simulink model "LQR"  (R2021b)
settings: Solver=VariableStepAuto  StartTime=0.0  StopTime=20  RelTol=1e-3
model workspace (MAT data in the model file):
  L = 0.2
values from neighbouring files (symbols this model uses):
  g = 9.81    [simConstants.m]
  K = lqr(A,B,Q,R,0)    [simConstants.m]
  theta0 = deg2rad(5)    [simConstants.m]
  Ts = 50e-6    (= 5e-05)    [simConstants.m]
libraries: simulink_extras x1
settings Model: Creator=logan  LastModifiedBy=logan

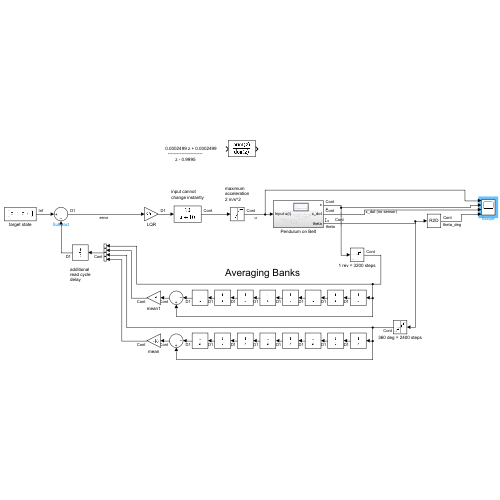
[thumbnail: Simulink's stored preview of the top-level diagram]
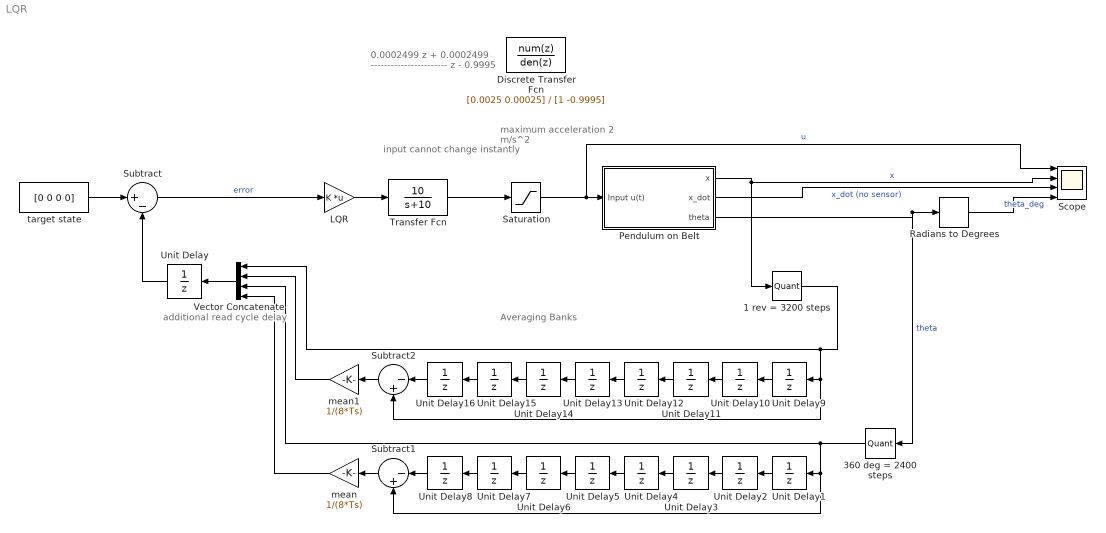
== system LQR ==
  note: 0.0002499 z + 0.0002499
      |   -----------------------
      |         z - 0.9995
  note: Averaging Banks
  note: input cannot
      | change instantly
  note: maximum
      | acceleration
      | 2 m/s^2
  note: additional
      | read cycle
      | delay
  1 rev = 3200 steps : Quantizer  QuantizationInterval=2*pi*0.006/3200
  360 deg = 2400 steps : Quantizer  QuantizationInterval=2*pi/2400
  Discrete Transfer Fcn : DiscreteTransferFcn  Numerator=[0.0025 0.00025]  Denominator=[1 -0.9995]
  LQR : Gain  Gain=K  Multiplication=Matrix(K*u)
  Pendulum on Belt : Subsystem
  Radians to Degrees : simulink_extras/Transformations/Radians to Degrees
  Saturation : Saturate  UpperLimit=2  LowerLimit=-2
  Scope : Scope  NumInputPorts=4
  Subtract : Sum  Inputs=|+-
  Subtract1 : Sum  Inputs=|-+
  Subtract2 : Sum  Inputs=|-+
  Transfer Fcn : TransferFcn  Numerator=[10]  Denominator=[1 10]
  Unit Delay{,1..16} (17 alike) : UnitDelay  SampleTime=Ts  HasFrameUpgradeWarning=on
  Vector Concatenate : Concatenate  NumInputs=4
  mean : Gain  Gain=1/(8*Ts)
  mean1 : Gain  Gain=1/(8*Ts)
  target state : Constant  Value=[0 0 0 0]  OutDataTypeStr=Inherit: Inherit via back propagation
  wires:
  Pendulum on Belt/1(x) -> Scope/2, 1 rev = 3200 steps/1  "x"
  Pendulum on Belt/3(theta) -> Radians to Degrees/1, 360 deg = 2400 steps/1  "theta"
  Radians to Degrees/1 -> Scope/4  "theta_deg"
  LQR/1 -> Transfer Fcn/1
  Subtract/1 -> LQR/1  "error"
  target state/1 -> Subtract/1
  Vector Concatenate/1 -> Unit Delay/1
  Unit Delay/1 -> Subtract/2
  360 deg = 2400 steps/1 -> Vector Concatenate/3, Unit Delay1/1, Subtract1/2
  Unit Delay1/1 -> Unit Delay2/1
  Unit Delay2/1 -> Unit Delay3/1
  Unit Delay3/1 -> Unit Delay4/1
  Unit Delay4/1 -> Unit Delay5/1
  Unit Delay5/1 -> Unit Delay6/1
  Unit Delay6/1 -> Unit Delay7/1
  Unit Delay7/1 -> Unit Delay8/1
  Unit Delay8/1 -> Subtract1/1
  Subtract1/1 -> mean/1
  mean/1 -> Vector Concatenate/4
  Saturation/1 -> Pendulum on Belt/1(Input u(t)), Scope/1  "u"
  Transfer Fcn/1 -> Saturation/1
  Unit Delay9/1 -> Unit Delay10/1
  Unit Delay15/1 -> Unit Delay16/1
  Unit Delay14/1 -> Unit Delay15/1
  Unit Delay13/1 -> Unit Delay14/1
  Unit Delay16/1 -> Subtract2/1
  Unit Delay12/1 -> Unit Delay13/1
  mean1/1 -> Vector Concatenate/2
  Unit Delay10/1 -> Unit Delay11/1
  1 rev = 3200 steps/1 -> Vector Concatenate/1, Unit Delay9/1, Subtract2/2
  Unit Delay11/1 -> Unit Delay12/1
  Subtract2/1 -> mean1/1
  Pendulum on Belt/2(x_dot) -> Scope/3  "x_dot (no sensor)"

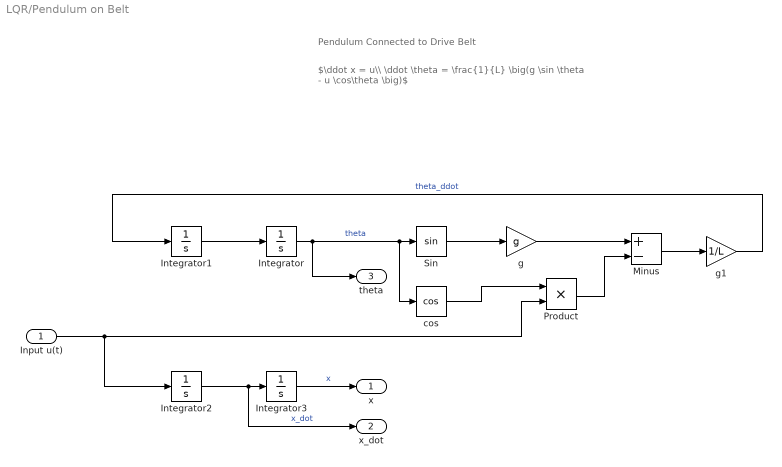
== system LQR/Pendulum on Belt ==
  note: Pendulum Connected to Drive Belt
  note: $\ddot x = u\\ \ddot \theta = \frac{1}{L} \big(g \sin \theta - u \cos\theta \big)$
  Input u(t) : Inport
  Integrator : Integrator  InitialCondition=theta0
  Integrator1 : Integrator
  Integrator2 : Integrator
  Integrator3 : Integrator
  Minus : Sum  Inputs=+-
  Product : Product
  Sin : Trigonometry
  cos : Trigonometry  Operator=cos
  g : Gain  Gain=g
  g1 : Gain  Gain=1/L
  x : Outport
  x_dot : Outport  Port=2
  theta : Outport  Port=3
  wires:
  Integrator/1 -> theta/1, cos/1, Sin/1  "theta"
  Integrator1/1 -> Integrator/1
  Input u(t)/1 -> Integrator2/1, Product/2
  g/1 -> Minus/1
  Sin/1 -> g/1
  cos/1 -> Product/1
  Integrator3/1 -> x/1  "x"
  Product/1 -> Minus/2
  Minus/1 -> g1/1
  g1/1 -> Integrator1/1  "theta_ddot"
  Integrator2/1 -> x_dot/1, Integrator3/1  "x_dot"
